simulink model "Boomerang_pitch_att_simulink"  (R2023a)
settings: Solver=ode4  StartTime=0.0  StopTime=t  FixedStep=dt  MaxStep=maxstep  MinStep=minstep*.1
values from neighbouring files (symbols this model uses):
  betaj = deg2rad(betaj)    [Boomerang4w_control.m]    (also in Boomerang_control_CoM.m; Boomerang_control_dihedral.m; Boomerang_control_gamma.m; Boomerang_control_pitch.m)
  c = 5e-2    (= 0.05)    [Boomerang4w_control.m]    (also in Boomerang_control_CoM.m = 0.0488; Boomerang_control_dihedral.m = 0.0488; Boomerang_control_gamma.m = 0.0488; Boomerang_control_pitch.m = 0.0488)
  CDdata = [x_CD, y_CD]    [Boomerang4w_control.m]    (also in Boomerang_control_CoM.m; Boomerang_control_dihedral.m; Boomerang_control_gamma.m; Boomerang_control_pitch.m)
  CLdata = [x_CL, y_CL]    [Boomerang4w_control.m]    (also in Boomerang_control_CoM.m; Boomerang_control_dihedral.m; Boomerang_control_gamma.m; Boomerang_control_pitch.m)
  CMdata = [x_CM, y_CM]    [Boomerang4w_control.m]    (also in Boomerang_control_CoM.m; Boomerang_control_dihedral.m; Boomerang_control_gamma.m; Boomerang_control_pitch.m)
  dt = 2e-4    (= 0.0002)    [Boomerang4w_control.m]    (also in Boomerang_control_CoM.m; Boomerang_control_dihedral.m; Boomerang_control_gamma.m; Boomerang_control_pitch.m)
  dt_con = 1/f_con    (= 0.001)    [Boomerang4w_control.m]
  Eul0 = [0; 0; 0]    [Boomerang4w_control.m]    (also in Boomerang_control_CoM.m; Boomerang_control_dihedral.m; Boomerang_control_gamma.m; Boomerang_control_pitch.m)
  g = 9.81    [Boomerang4w_control.m]    (also in Boomerang_control_CoM.m; Boomerang_control_dihedral.m; Boomerang_control_gamma.m; Boomerang_control_pitch.m)
  gamma = deg2rad(gamma)    [Boomerang4w_control.m]    (also in Boomerang_control_CoM.m; Boomerang_control_dihedral.m; Boomerang_control_gamma.m; Boomerang_control_pitch.m)
  invTI0 = transpose(TI0)    [Boomerang4w_control.m]    (also in Boomerang_control_CoM.m; Boomerang_control_dihedral.m; Boomerang_control_gamma.m; Boomerang_control_pitch.m)
  J = J + (Ji(:,:,i))    [Boomerang4w_control.m]    (also in Boomerang_control_CoM.m = diag(diag(J)); Boomerang_control_dihedral.m = diag(diag(J)); Boomerang_control_gamma.m = diag(diag(J)); Boomerang_control_pitch.m = diag(diag(J)))
  Jj = [ ... (first row only)    [Boomerang4w_control.m]    (also in Boomerang_control_CoM.m; Boomerang_control_dihedral.m; Boomerang_control_gamma.m; Boomerang_control_pitch.m)
  Kd = 0.    (= 0)    [Boomerang4w_control.m]    (also in Boomerang_control_CoM.m; Boomerang_control_dihedral.m; Boomerang_control_gamma.m; Boomerang_control_pitch.m)
  Kd_roll = 0    [Boomerang4w_control.m]    (also in Boomerang_control_pitch.m = 0.004)
  Ki = 0.    (= 0)    [Boomerang4w_control.m]    (also in Boomerang_control_CoM.m; Boomerang_control_dihedral.m; Boomerang_control_gamma.m; Boomerang_control_pitch.m)
  Ki_roll = 0    [Boomerang4w_control.m]    (also in Boomerang_control_pitch.m = 15)
  Kp = .0    (= 0)    [Boomerang4w_control.m]    (also in Boomerang_control_CoM.m; Boomerang_control_dihedral.m; Boomerang_control_gamma.m; Boomerang_control_pitch.m)
  Kp_roll = 0    [Boomerang4w_control.m]    (also in Boomerang_control_pitch.m = 2)
  l_integrate = linspace(0,l_blade,n)    [Boomerang4w_control.m]    (also in Boomerang_control_CoM.m; Boomerang_control_dihedral.m; Boomerang_control_gamma.m; Boomerang_control_pitch.m)
  LAMBDAj = deg2rad(LAMBDAj)    [Boomerang4w_control.m]    (also in Boomerang_control_CoM.m; Boomerang_control_dihedral.m; Boomerang_control_gamma.m; Boomerang_control_pitch.m)
  m = 200e-3    (= 0.2)    [Boomerang4w_control.m]    (also in Boomerang_control_CoM.m = 0.13; Boomerang_control_dihedral.m = 0.13; Boomerang_control_gamma.m = 0.13; Boomerang_control_pitch.m = 0.13)
  n = n + 1    (= 51)    [Boomerang4w_control.m]    (also in Boomerang_control_CoM.m; Boomerang_control_dihedral.m; Boomerang_control_gamma.m; Boomerang_control_pitch.m)
  nw = 4    [Boomerang4w_control.m]    (also in Boomerang_control_CoM.m = 2; Boomerang_control_dihedral.m = 2; Boomerang_control_gamma.m = 2; Boomerang_control_pitch.m = 2)
  omega0 = [0; 0; 10*pi*2]    [Boomerang4w_control.m]    (also in Boomerang_control_CoM.m; Boomerang_control_dihedral.m; Boomerang_control_gamma.m; Boomerang_control_pitch.m)
  PHI_des = deg2rad(PHI_des)    [Boomerang4w_control.m]    (also in Boomerang_control_pitch.m)
  R_pos0 = [0; 0; 1.5]    [Boomerang4w_control.m]    (also in Boomerang_control_CoM.m; Boomerang_control_dihedral.m; Boomerang_control_gamma.m; Boomerang_control_pitch.m)
  rho = 1.22    [Boomerang4w_control.m]    (also in Boomerang_control_CoM.m; Boomerang_control_dihedral.m; Boomerang_control_gamma.m; Boomerang_control_pitch.m)
  S = pi*R^2    (= 0.196349540849)    [Boomerang4w_control.m]    (also in Boomerang_control_CoM.m = 0.228; Boomerang_control_dihedral.m = 0.228; Boomerang_control_gamma.m = 0.228; Boomerang_control_pitch.m = 0.228)
  servo_rpm = deg2rad(servo_rpm)    [Boomerang4w_control.m]    (also in Boomerang_control_dihedral.m; Boomerang_control_gamma.m; Boomerang_control_pitch.m; Pitch_control_trajectory_wy.mat = 8.72664625997)
  theta_sat = deg2rad(theta_sat)    [Boomerang4w_control.m]    (also in Boomerang_control_pitch.m)
  TI0 = RI01*RI02*RI03    [Boomerang4w_control.m]    (also in Boomerang_control_CoM.m; Boomerang_control_dihedral.m; Boomerang_control_gamma.m; Boomerang_control_pitch.m)
  u0 = TI0*U0    [Boomerang4w_control.m]    (also in Boomerang_control_CoM.m; Boomerang_control_dihedral.m; Boomerang_control_gamma.m; Boomerang_control_pitch.m)
  v_wind = [-1; 0; 0]    [Boomerang4w_control.m]    (also in Boomerang_control_CoM.m = [0; 0; 0]; Boomerang_control_dihedral.m = [0; 0; 0]; Boomerang_control_gamma.m = [0; 0; 0]; Boomerang_control_pitch.m = [0; 0; 0])
  x_ac = zeros(3,nw)    [Boomerang4w_control.m]    (also in Boomerang_control_CoM.m = 0.061; Boomerang_control_dihedral.m = 0.061; Boomerang_control_gamma.m = 0.061; Boomerang_control_pitch.m = 0.061)
  X_des = [x_des, y_des]    [Boomerang4w_control.m]    (also in Boomerang_control_CoM.m; Boomerang_control_dihedral.m; Boomerang_control_gamma.m; Boomerang_control_pitch.m)
settings Model: Creator=dsantis  LastModifiedBy=dsantis

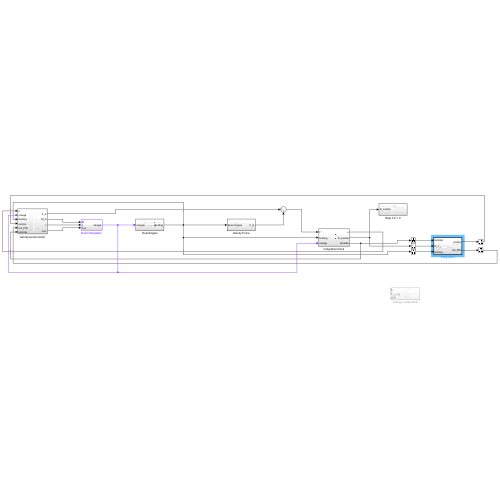
[thumbnail: Simulink's stored preview of the top-level diagram]
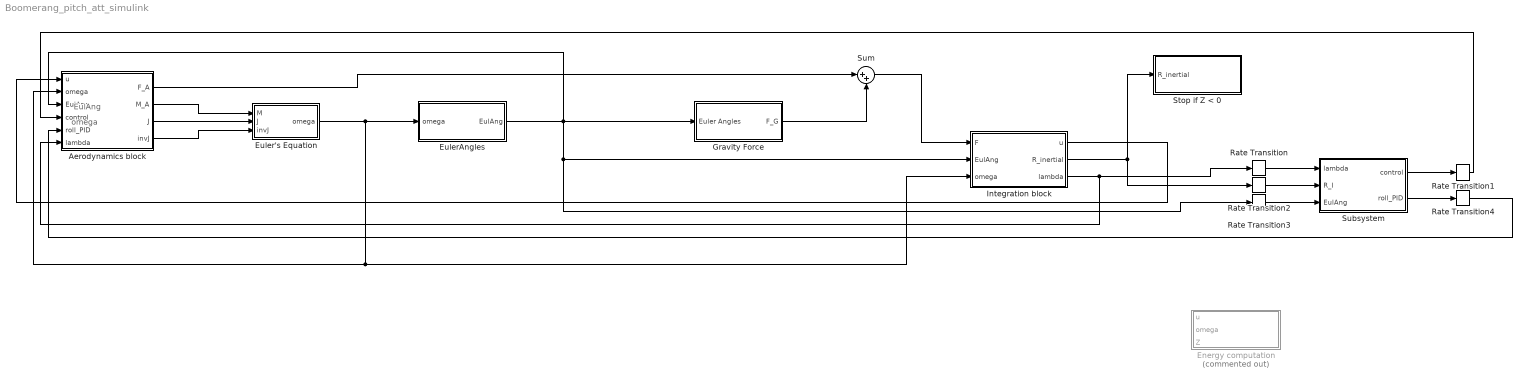
== system Boomerang_pitch_att_simulink ==
  note: omega
  note: EulAng
  Aerodynamics block : Subsystem
  Energy computation : Subsystem  Commented=on
  Euler's Equation : Subsystem
  EulerAngles : Subsystem
  Gravity Force : Subsystem
  Integration block : Subsystem
  Rate Transition : RateTransition  InitialCondition=dt  OutPortSampleTime=dt_con
  Rate Transition1 : RateTransition  InitialCondition=dt_con  OutPortSampleTime=dt
  Rate Transition2 : RateTransition  InitialCondition=dt  OutPortSampleTime=dt_con
  Rate Transition3 : RateTransition  InitialCondition=dt  OutPortSampleTime=dt_con
  Rate Transition4 : RateTransition  InitialCondition=dt_con  OutPortSampleTime=dt
  Stop if Z < 0 : Subsystem
  Subsystem : Subsystem  TreatAsAtomicUnit=on
  Sum : Sum  Inputs=|++
  wires:
  Aerodynamics block/1(F_A) -> Sum/1
  Euler's Equation/1(omega) -> Aerodynamics block/2(omega), Integration block/3(omega), EulerAngles/1(omega)
  Sum/1 -> Integration block/1(F)
  Gravity Force/1(F_G) -> Sum/2
  Aerodynamics block/2(M_A) -> Euler's Equation/1(M)
  EulerAngles/1(EulAng) -> Rate Transition3/1, Integration block/2(EulAng), Gravity Force/1(Euler Angles), Aerodynamics block/3(EulAng)
  Integration block/2(R_inertial) -> Rate Transition2/1, Stop if Z < 0/1(R_inertial)
  Aerodynamics block/3(J) -> Euler's Equation/2(J)
  Aerodynamics block/4(invJ) -> Euler's Equation/3(invJ)
  Rate Transition/1 -> Subsystem/1(lambda)
  Rate Transition1/1 -> Aerodynamics block/4(control)
  Rate Transition4/1 -> Aerodynamics block/5(roll_PID)
  Rate Transition2/1 -> Subsystem/2(R_I)
  Rate Transition3/1 -> Subsystem/3(EulAng)
  Integration block/1(u) -> Aerodynamics block/1(u)
  Subsystem/1(control) -> Rate Transition1/1
  Subsystem/2(roll_PID) -> Rate Transition4/1
  Integration block/3(lambda) -> Aerodynamics block/6(lambda), Rate Transition/1

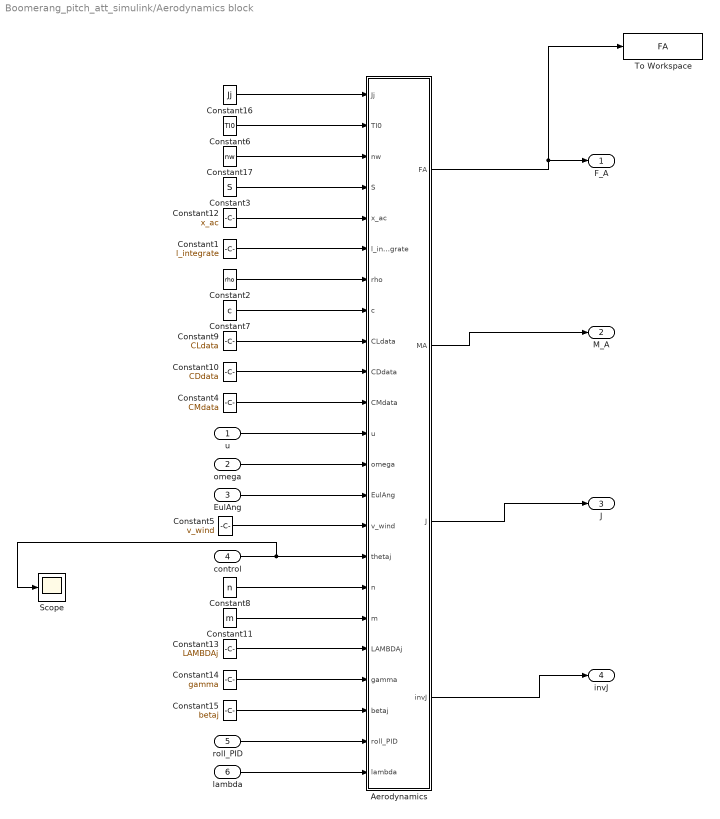
== system Boomerang_pitch_att_simulink/Aerodynamics block ==
  u : Inport
  omega : Inport  Port=2
  EulAng : Inport  Port=3
  control : Inport  Port=4
  roll_PID : Inport  Port=5
  lambda : Inport  Port=6
  Aerodynamics : MATLAB Function  TreatAsAtomicUnit=on
  Constant1 : Constant  Value=l_integrate
  Constant10 : Constant  Value=CDdata
  Constant11 : Constant  Value=m
  Constant12 : Constant  Value=x_ac
  Constant13 : Constant  Value=LAMBDAj
  Constant14 : Constant  Value=gamma
  Constant15 : Constant  Value=betaj
  Constant16 : Constant  Value=Jj
  Constant17 : Constant  Value=nw
  Constant2 : Constant  Value=rho
  Constant3 : Constant  Value=S
  Constant4 : Constant  Value=CMdata
  Constant5 : Constant  Value=v_wind
  Constant6 : Constant  Value=TI0
  Constant7 : Constant  Value=c
  Constant8 : Constant  Value=n
  Constant9 : Constant  Value=CLdata
  Scope : Scope
  To Workspace : ToWorkspace  VariableName=FA  SampleTime=-1
  F_A : Outport
  M_A : Outport  Port=2
  J : Outport  Port=3
  invJ : Outport  Port=4
  wires:
  u/1 -> Aerodynamics/12(u)
  Constant2/1 -> Aerodynamics/7(rho)
  Constant9/1 -> Aerodynamics/9(CLdata)
  Constant10/1 -> Aerodynamics/10(CDdata)
  Constant1/1 -> Aerodynamics/6(l_integrate)
  Constant7/1 -> Aerodynamics/8(c)
  omega/1 -> Aerodynamics/13(omega)
  Constant12/1 -> Aerodynamics/5(x_ac)
  Constant17/1 -> Aerodynamics/3(nw)
  Constant3/1 -> Aerodynamics/4(S)
  Aerodynamics/1(FA) -> To Workspace/1, F_A/1
  Constant4/1 -> Aerodynamics/11(CMdata)
  Aerodynamics/2(MA) -> M_A/1
  EulAng/1 -> Aerodynamics/14(EulAng)
  control/1 -> Scope/1, Aerodynamics/16(thetaj)
  Constant5/1 -> Aerodynamics/15(v_wind)
  Constant6/1 -> Aerodynamics/2(TI0)
  Constant8/1 -> Aerodynamics/17(n)
  Aerodynamics/3(J) -> J/1
  Aerodynamics/4(invJ) -> invJ/1
  Constant11/1 -> Aerodynamics/18(m)
  Constant13/1 -> Aerodynamics/19(LAMBDAj)
  Constant14/1 -> Aerodynamics/20(gamma)
  Constant15/1 -> Aerodynamics/21(betaj)
  roll_PID/1 -> Aerodynamics/22(roll_PID)
  Constant16/1 -> Aerodynamics/1(Jj)
  lambda/1 -> Aerodynamics/23(lambda)

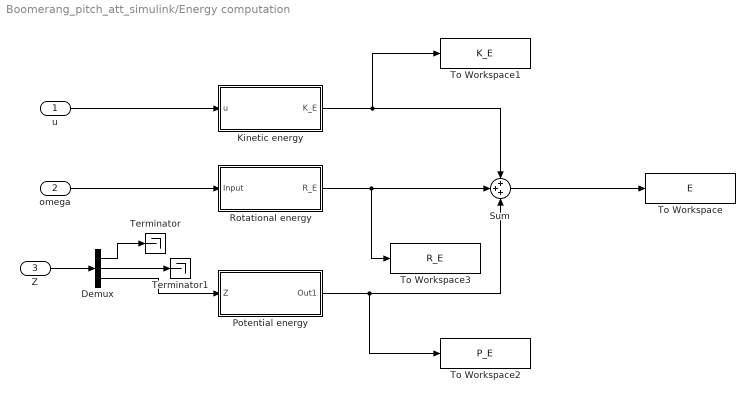
== system Boomerang_pitch_att_simulink/Energy computation ==
  u : Inport
  omega : Inport  Port=2
  Z : Inport  Port=3
  Demux : Demux  Outputs=3
  Kinetic energy : Subsystem
  Potential energy : Subsystem
  Rotational energy : Subsystem
  Sum : Sum  Inputs=+++
  Terminator : Terminator
  Terminator1 : Terminator
  To Workspace : ToWorkspace  VariableName=E  SaveFormat=Timeseries  SampleTime=-1
  To Workspace1 : ToWorkspace  VariableName=K_E  SaveFormat=Timeseries  SampleTime=-1
  To Workspace2 : ToWorkspace  VariableName=P_E  SaveFormat=Timeseries  SampleTime=-1
  To Workspace3 : ToWorkspace  VariableName=R_E  SaveFormat=Timeseries  SampleTime=-1
  wires:
  u/1 -> Kinetic energy/1(u)
  omega/1 -> Rotational energy/1(Input)
  Z/1 -> Demux/1
  Demux/3 -> Potential energy/1(Z)
  Demux/1 -> Terminator/1
  Demux/2 -> Terminator1/1
  Kinetic energy/1(K_E) -> To Workspace1/1, Sum/1
  Rotational energy/1(R_E) -> To Workspace3/1, Sum/2
  Potential energy/1(Out1) -> To Workspace2/1, Sum/3
  Sum/1 -> To Workspace/1

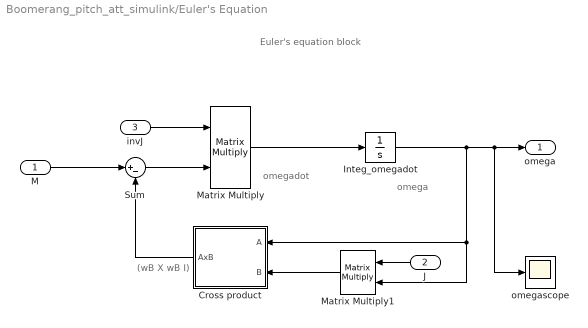
== system Boomerang_pitch_att_simulink/Euler's Equation ==
  note: Euler's equation block
  note: (wB X wB I)
  note: omega
  note: omegadot
  M : Inport
  J : Inport  Port=2
  invJ : Inport  Port=3
  Cross product : Subsystem
  Integ_omegadot : Integrator  InitialCondition=omega0
  Matrix Multiply : Product  Multiplication=Matrix(*)
  Matrix Multiply1 : Product  Multiplication=Matrix(*)
  Sum : Sum  Inputs=|+-
  omegascope : Scope
  omega : Outport  VectorParamsAs1DForOutWhenUnconnected=off
  wires:
  Integ_omegadot/1 -> Cross product/1(A), Matrix Multiply1/2, omegascope/1, omega/1
  Matrix Multiply1/1 -> Cross product/2(B)
  M/1 -> Sum/1
  Sum/1 -> Matrix Multiply/2
  Matrix Multiply/1 -> Integ_omegadot/1
  Cross product/1(AxB) -> Sum/2
  invJ/1 -> Matrix Multiply/1
  J/1 -> Matrix Multiply1/1

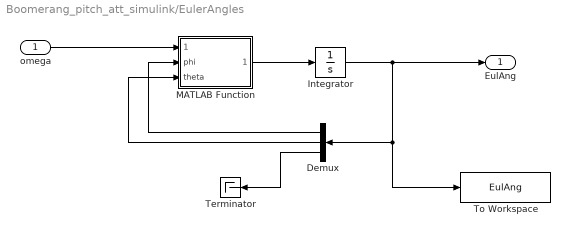
== system Boomerang_pitch_att_simulink/EulerAngles ==
  omega : Inport
  Demux : Demux  Outputs=3
  Integrator : Integrator  InitialCondition=Eul0
  MATLAB Function : MATLAB Function  TreatAsAtomicUnit=on
  Terminator : Terminator
  To Workspace : ToWorkspace  VariableName=EulAng  SampleTime=-1
  EulAng : Outport
  wires:
  omega/1 -> MATLAB Function/1(omega)
  MATLAB Function/1(EulRate) -> Integrator/1
  Integrator/1 -> Demux/1, To Workspace/1, EulAng/1
  Demux/1 -> MATLAB Function/2(phi)
  Demux/2 -> MATLAB Function/3(theta)
  Demux/3 -> Terminator/1

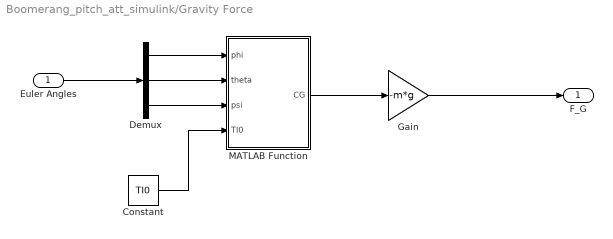
== system Boomerang_pitch_att_simulink/Gravity Force ==
  Euler Angles : Inport
  Constant : Constant  Value=TI0
  Demux : Demux  Outputs=3
  Gain : Gain  Gain=-m*g
  MATLAB Function : MATLAB Function  TreatAsAtomicUnit=on
  F_G : Outport
  wires:
  Gain/1 -> F_G/1
  Demux/3 -> MATLAB Function/3(psi)
  Demux/2 -> MATLAB Function/2(theta)
  Demux/1 -> MATLAB Function/1(phi)
  MATLAB Function/1(CG) -> Gain/1
  Euler Angles/1 -> Demux/1
  Constant/1 -> MATLAB Function/4(TI0)

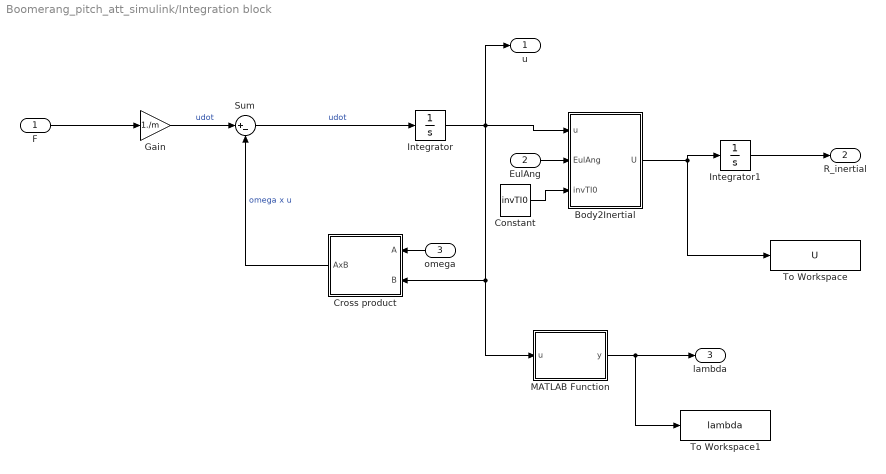
== system Boomerang_pitch_att_simulink/Integration block ==
  F : Inport
  EulAng : Inport  Port=2
  omega : Inport  Port=3
  Body2Inertial : MATLAB Function  TreatAsAtomicUnit=on
  Constant : Constant  Value=invTI0
  Cross product : Subsystem
  Gain : Gain  Gain=1./m
  Integrator : Integrator  InitialCondition=u0
  Integrator1 : Integrator  InitialCondition=R_pos0
  MATLAB Function : MATLAB Function  TreatAsAtomicUnit=on
  Sum : Sum  Inputs=|+-
  To Workspace : ToWorkspace  VariableName=U  SampleTime=-1
  To Workspace1 : ToWorkspace  VariableName=lambda  SampleTime=-1
  u : Outport
  R_inertial : Outport  Port=2
  lambda : Outport  Port=3
  wires:
  Cross product/1(AxB) -> Sum/2  "omega x u"
  Integrator1/1 -> R_inertial/1
  Gain/1 -> Sum/1  "udot"
  EulAng/1 -> Body2Inertial/2(EulAng)
  Constant/1 -> Body2Inertial/3(invTI0)
  F/1 -> Gain/1
  Body2Inertial/1(U) -> Integrator1/1, To Workspace/1
  Sum/1 -> Integrator/1  "udot"
  omega/1 -> Cross product/1(A)
  MATLAB Function/1(y) -> To Workspace1/1, lambda/1
  Integrator/1 -> MATLAB Function/1(u), Cross product/2(B), Body2Inertial/1(u), u/1

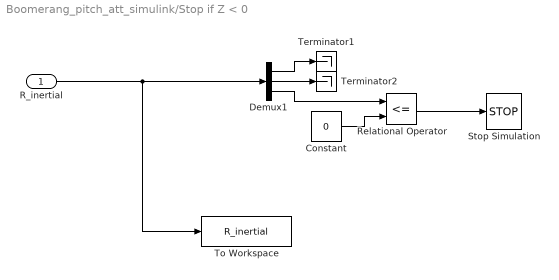
== system Boomerang_pitch_att_simulink/Stop if Z < 0 ==
  R_inertial : Inport
  Constant : Constant  Value=0
  Demux1 : Demux  Outputs=3
  Relational Operator : RelationalOperator  Operator=<=  OutDataTypeStr=boolean  RndMeth=Simplest  InputSameDT=off
  Stop Simulation : Stop
  Terminator1 : Terminator
  Terminator2 : Terminator
  To Workspace : ToWorkspace  VariableName=R_inertial  SampleTime=-1
  wires:
  R_inertial/1 -> To Workspace/1, Demux1/1
  Demux1/1 -> Terminator1/1
  Demux1/3 -> Relational Operator/1
  Demux1/2 -> Terminator2/1
  Constant/1 -> Relational Operator/2
  Relational Operator/1 -> Stop Simulation/1

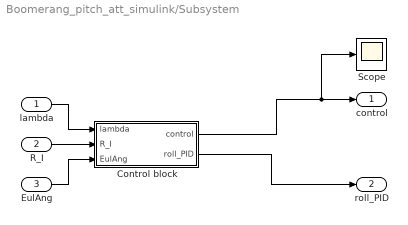
== system Boomerang_pitch_att_simulink/Subsystem ==
  lambda : Inport
  R_I : Inport  Port=2
  EulAng : Inport  Port=3
  Control block : Subsystem
  Scope : Scope
  control : Outport
  roll_PID : Outport  Port=2
  wires:
  lambda/1 -> Control block/1(lambda)
  R_I/1 -> Control block/2(R_I)
  EulAng/1 -> Control block/3(EulAng)
  Control block/2(roll_PID) -> roll_PID/1
  Control block/1(control) -> Scope/1, control/1

== system Boomerang_pitch_att_simulink/Energy computation/Kinetic energy ==
  u : Inport
  Gain : Gain  Gain=0.5*m
  Norm : MATLAB Function  TreatAsAtomicUnit=on
  K_E : Outport
  wires:
  u/1 -> Norm/1(u)
  Norm/1(y) -> Gain/1
  Gain/1 -> K_E/1

== system Boomerang_pitch_att_simulink/Energy computation/Potential energy ==
  Z : Inport
  Gain : Gain  Gain=m*g
  Out1 : Outport
  wires:
  Z/1 -> Gain/1
  Gain/1 -> Out1/1

== system Boomerang_pitch_att_simulink/Energy computation/Rotational energy ==
  Input : Inport
  Dot Product : DotProduct  OutDataTypeStr=Inherit: Inherit via internal rule
  Gain : Gain  Gain=0.5*J  Multiplication=Matrix(u*K)
  R_E : Outport
  wires:
  Input/1 -> Dot Product/2, Gain/1
  Gain/1 -> Dot Product/1
  Dot Product/1 -> R_E/1

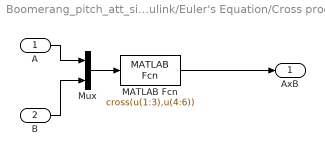
== system Boomerang_pitch_att_simulink/Euler's Equation/Cross product ==
  A : Inport
  B : Inport  Port=2
  MATLAB Fcn : MATLABFcn  MATLABFcn=cross(u(1:3),u(4:6))
  Mux : Mux  Inputs=2
  AxB : Outport  VectorParamsAs1DForOutWhenUnconnected=off
  wires:
  A/1 -> Mux/1
  B/1 -> Mux/2
  Mux/1 -> MATLAB Fcn/1
  MATLAB Fcn/1 -> AxB/1

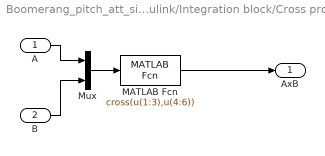
== system Boomerang_pitch_att_simulink/Integration block/Cross product ==
  A : Inport
  B : Inport  Port=2
  MATLAB Fcn : MATLABFcn  MATLABFcn=cross(u(1:3),u(4:6))
  Mux : Mux  Inputs=2
  AxB : Outport  VectorParamsAs1DForOutWhenUnconnected=off
  wires:
  A/1 -> Mux/1
  B/1 -> Mux/2
  Mux/1 -> MATLAB Fcn/1
  MATLAB Fcn/1 -> AxB/1

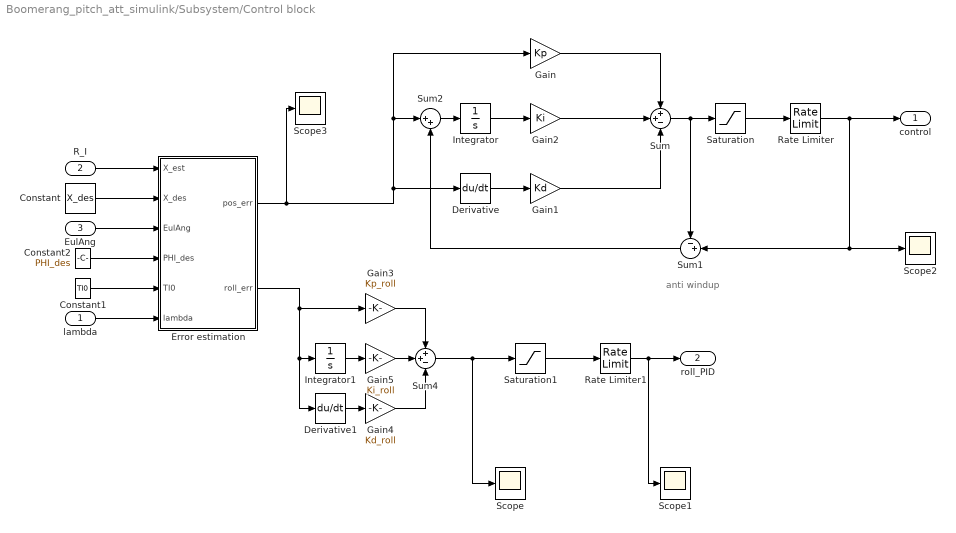
== system Boomerang_pitch_att_simulink/Subsystem/Control block ==
  note: anti windup
  lambda : Inport
  R_I : Inport  Port=2
  EulAng : Inport  Port=3
  Constant : Constant  Value=X_des
  Constant1 : Constant  Value=TI0
  Constant2 : Constant  Value=PHI_des
  Derivative : Derivative
  Derivative1 : Derivative
  Error estimation : MATLAB Function  TreatAsAtomicUnit=on
  Gain : Gain  Gain=Kp
  Gain1 : Gain  Gain=Kd
  Gain2 : Gain  Gain=Ki
  Gain3 : Gain  Gain=Kp_roll
  Gain4 : Gain  Gain=Kd_roll
  Gain5 : Gain  Gain=Ki_roll
  Integrator : Integrator  UpperSaturationLimit=pi/Ki  LowerSaturationLimit=-pi/Ki
  Integrator1 : Integrator
  Rate Limiter : RateLimiter  RisingSlewLimit=servo_rpm  FallingSlewLimit=-servo_rpm  SampleTimeMode=inherited
  Rate Limiter1 : RateLimiter  RisingSlewLimit=servo_rpm  FallingSlewLimit=-servo_rpm  SampleTimeMode=inherited
  Saturation : Saturate  UpperLimit=theta_sat  LowerLimit=-theta_sat
  Saturation1 : Saturate  UpperLimit=theta_sat  LowerLimit=-theta_sat
  Scope{,1..3} (4 alike) : Scope
  Sum : Sum  Inputs=++-
  Sum1 : Sum  Inputs=-+|
  Sum2 : Sum  Inputs=|++
  Sum4 : Sum  Inputs=++-
  control : Outport
  roll_PID : Outport  Port=2
  wires:
  R_I/1 -> Error estimation/1(X_est)
  Constant/1 -> Error estimation/2(X_des)
  Error estimation/1(pos_err) -> Scope3/1, Gain/1, Sum2/1, Derivative/1
  Gain/1 -> Sum/1
  Derivative/1 -> Gain1/1
  Gain1/1 -> Sum/3
  Saturation/1 -> Rate Limiter/1
  Rate Limiter/1 -> Scope2/1, Sum1/2, control/1
  Integrator/1 -> Gain2/1
  Gain2/1 -> Sum/2
  Sum2/1 -> Integrator/1
  Sum1/1 -> Sum2/2
  Sum/1 -> Saturation/1, Sum1/1
  lambda/1 -> Error estimation/6(lambda)
  EulAng/1 -> Error estimation/3(EulAng)
  Gain3/1 -> Sum4/1
  Constant2/1 -> Error estimation/4(PHI_des)
  Derivative1/1 -> Gain4/1
  Gain4/1 -> Sum4/3
  Integrator1/1 -> Gain5/1
  Error estimation/2(roll_err) -> Integrator1/1, Derivative1/1, Gain3/1
  Gain5/1 -> Sum4/2
  Constant1/1 -> Error estimation/5(TI0)
  Sum4/1 -> Saturation1/1, Scope/1
  Saturation1/1 -> Rate Limiter1/1
  Rate Limiter1/1 -> Scope1/1, roll_PID/1

== matlab function Boomerang_pitch_att_simulink/Subsystem/Control block/Error estimation ==
  settings: updateMethod=DISCRETE
  data: pos_err output; X_est input; X_des input; EulAng input; PHI_des input; TI0 input; lambda input; roll_err output
function [pos_err, roll_err] = fcn(X_est,X_des, EulAng, PHI_des, TI0, lambda)

phi = EulAng(1);
theta = EulAng(2);
psi = EulAng(3);

Tn = [cos(lambda) -sin(lambda) 0; sin(lambda) cos(lambda) 0; 0 0 1];

R01 = [1, 0, 0; 0, cos(phi), sin(phi); 0, -sin(phi), cos(phi)];
R02 = [cos(theta), 0, -sin(theta); 0, 1, 0; sin(theta), 0, cos(theta)];
R03 = [cos(psi), sin(psi), 0; -sin(psi), cos(psi), 0; 0, 0, 1];

T0 = R01*R02*R03;

TI = Tn*T0*TI0;
THETA = -asin(TI(1,3));
% PSI = acos( TI(1,1)/cos(THETA) );
PHI = acos( TI(3,3)/cos(THETA) );

% Find which desired trajectory point is nearest to the boomerang and
% compute the error. 
[err_vec, i] = min(vecnorm([X_est(1), X_est(2)] - X_des,2,2));

% Figure out if you are to the left or to the right of the desired
% trajectory in order to determine the sign of the error and follow with
% the proper control maneuver
err_sign = sign(norm([X_est(1), X_est(2)]) - norm([X_des(i,1), X_des(i,2)]));

roll_err = PHI_des - PHI;
pos_err = err_sign*err_vec;
if err_sign == -1
        pos_err = 0;
end


end

== matlab function Boomerang_pitch_att_simulink/Energy computation/Kinetic energy/Norm ==
  data: u input; y output
function y = fcn(u)

y = norm(u)^2;

== matlab function Boomerang_pitch_att_simulink/Integration block/MATLAB Function ==
  data: u input; y output
function y = fcn(u)
    
y = -atan2(u(2),u(1));

== matlab function Boomerang_pitch_att_simulink/Aerodynamics block/Aerodynamics ==
  settings: updateMethod=DISCRETE
  data: Jj input; TI0 input; nw input; S input; x_ac input; l_integrate input; rho input; c input; CLdata input; CDdata input; CMdata input; u input; omega input; EulAng input; v_wind input; FA output; thetaj input; MA output; n input; J output; invJ output; m input; LAMBDAj input; gamma input; betaj input; roll_PID input; lambda input
function [FA, MA, J, invJ] = fcn(Jj, TI0, nw, S, x_ac, l_integrate, rho, c, CLdata, CDdata, CMdata,u, omega, EulAng, v_wind, thetaj, n, m, LAMBDAj, gamma, betaj, roll_PID, lambda)
phi = EulAng(1);
theta = EulAng(2);
psi = EulAng(3);

R01 = [1, 0, 0; 0, cos(phi), sin(phi); 0, -sin(phi), cos(phi)];
R02 = [cos(theta), 0, -sin(theta); 0, 1, 0; sin(theta), 0, cos(theta)];
R03 = [cos(psi), sin(psi), 0; -sin(psi), cos(psi), 0; 0, 0, 1];
T0 = R01*R02*R03;

Tj = zeros(3,3, nw);
invTj = zeros(3,3,nw);

for i = 0:(nw-1)
Rj1 = [1, 0, 0; 0, cos(betaj), sin(betaj); 0, -sin(betaj), cos(betaj)];
    Rj2 = [cos(thetaj), 0, -sin(thetaj);0, 1, 0; sin(thetaj), 0, cos(thetaj)];
    Rj3 = [cos(LAMBDAj-pi/2 + gamma*i), sin(LAMBDAj-pi/2 + gamma*i), 0; ...
        -sin(LAMBDAj-pi/2 + gamma*i), cos(LAMBDAj-pi/2+ gamma*i), 0;0, 0, 1];
    Tj(:,:,i+1) = Rj2*Rj1*Rj3;
    invTj(:,:,i+1) = transpose(Tj(:,:,i+1));
end
Ji = zeros(3,3,nw);
J = zeros(3);
for i = 1:nw
    Ji(:,:,i) = invTj(:,:,i)*Jj*Tj(:,:,i);
    J = J + (Ji(:,:,i));
end
% J = diag(diag(J));

invJ = inv(J);
r = l_integrate./l_integrate(end);

persistent flag v_bar
if isempty(flag)
    flag = false;
    v_bar = 0;
end

% Piecewise linear fit for CL
C_L = @(alpha) interp1(CLdata(:,1), CLdata(:,2), alpha, 'linear', 'extrap');

% Piecewise linear fit for CD
C_D = @(alpha) interp1(CDdata(:,1), CDdata(:,2), alpha, 'linear', 'extrap');

 % Piecewise linear fit for CM
C_M = @(alpha) interp1(CMdata(:,1), CMdata(:,2), alpha, 'linear', 'extrap');

FA = [0; 0; 0];
MA = [0;0;0];

for i = 1:nw
    % Computing induced velocity considering linear variation along the
    % longitudinal direction
    kx = 1.5;
    v_ind = [zeros(size(l_integrate)), zeros(size(l_integrate)), v_bar*(1+kx*cos(lambda + gamma*(i-1))*r)]';

    rA = x_ac(:,i).*ones(3,n) + invTj(:,:,i)*[zeros(1,n); l_integrate'; zeros(1,n)];
    
    w = Tj(:,:,i)*( (-u -cross(omega.*ones(3,n), rA)) + v_ind + T0*TI0*v_wind);
    alpha = (atan2(w(3,:),w(1,:))) + thetaj + roll_PID*cos(lambda +  gamma*(i-1) - pi);
    
    % Computing the tip-loss factor F
    f = abs(nw/2.*(1-r')./(r'.*alpha));
    F =2/pi*acos(exp(-f));
    w2 = w(1,:).^2 + w(3,:).^2;
    
    l = (0.5*rho*c).*w2.*C_L(alpha);
    d = (0.5*rho*c).*w2.*C_D(alpha);
    m_eta = (0.5*rho*c^2).*w2.*C_M(alpha);

    int_funx = F.*(-l.*sin(alpha) + d.*cos(alpha));
    int_funz = (l.*cos(alpha) + d.*sin(alpha));
    
    % int_funMx = (l.*cos(alpha) + d.*sin(alpha)).*l_integrate';
    funM = cross([zeros(1,n); l_integrate'; zeros(1,n)], [int_funx; zeros(1,n); int_funz]);
    int_funMx = funM(1,:);
    int_funMy = m_eta; 
    int_funMz = funM(3,:);
 
    FxjA = trapz(l_integrate,int_funx);
    FzjA = trapz(l_integrate,int_funz);

    MxjA = trapz(l_integrate,int_funMx);
    MyjA = trapz(l_integrate,int_funMy);
    MzjA = trapz(l_integrate,int_funMz);

    FjA = [FxjA; 0; FzjA];
    FA = FA + invTj(:,:,i)*FjA;

    MjA = [MxjA'; MyjA; MzjA];
    MA = MA + invTj(:,:,i)*MjA + cross(x_ac(:,i), invTj(:,:,i)*FjA);
end
f = @(v_ind) v_ind - FA(3)/(2*rho*S*sqrt(norm([u(1) u(2)])^2 + (u(3)-v_ind)^2));
v_bar = fzero(f,0);

== matlab function Boomerang_pitch_att_simulink/Gravity Force/MATLAB Function ==
  data: phi input; theta input; psi input; CG output; TI0 input
function CG = fcn(phi, theta, psi, TI0)
R01 = [
    1, 0, 0;
    0, cos(phi), sin(phi);
    0, -sin(phi), cos(phi)
    ];
R02 = [
    cos(theta), 0, -sin(theta);
    0, 1, 0;
    sin(theta), 0, cos(theta)
];
R03 = [
    cos(psi), sin(psi), 0;
    -sin(psi), cos(psi), 0;
    0, 0, 1
];
T0 = R01*R02*R03;

CG = T0*TI0*[0; 0; 1];

== matlab function Boomerang_pitch_att_simulink/Integration block/Body2Inertial ==
  data: u input; U output; EulAng input; invTI0 input
function U = fcn(u, EulAng, invTI0)
phi = EulAng(1);
theta = EulAng(2);
psi = EulAng(3);

R01 = [
    1, 0, 0;
    0, cos(phi), sin(phi);
    0, -sin(phi), cos(phi)
    ];
R02 = [
    cos(theta), 0, -sin(theta);
    0, 1, 0;
    sin(theta), 0, cos(theta)
];
R03 = [
    cos(psi), sin(psi), 0;
    -sin(psi), cos(psi), 0;
    0, 0, 1
];
T0 = R01*R02*R03;
invT0 = transpose(T0);
U = invTI0*invT0*u;

== matlab function Boomerang_pitch_att_simulink/EulerAngles/MATLAB Function ==
  data: omega input; EulRate output; phi input; theta input
function EulRate = fcn(omega, phi, theta)

phidot = omega(1) + omega(2)*sin(phi)*tan(theta) + omega(3)*cos(phi)*tan(theta);
thetadot = omega(2)*cos(phi) - omega(3)*sin(phi);
psidot = omega(2)*sin(phi)/cos(theta) + omega(3)*cos(phi)/cos(theta);

EulRate = [phidot; thetadot; psidot];
